simulink model "Rate_Transition_Idea"  (R2013b)
settings: Solver=ode45  StartTime=0.0  StopTime=10.0  RelTol=1e-3
settings Model: Creator=Eduardo  LastModifiedBy=Eduardo

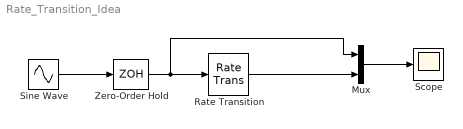
== system Rate_Transition_Idea ==
  Mux : Mux  Inputs=2
  Rate Transition : RateTransition  OutPortSampleTime=0.03
  Scope : Scope
  Sine Wave : Sin  SampleTime=0
  Zero-Order Hold : ZeroOrderHold  SampleTime=0.01
  wires:
  Sine Wave/1 -> Zero-Order Hold/1
  Zero-Order Hold/1 -> Mux/1, Rate Transition/1
  Mux/1 -> Scope/1
  Rate Transition/1 -> Mux/2
